simulink model "test_VirtualTestRig"  (R2021b)
settings: Solver=VariableStepAuto  StartTime=0.0  StopTime=10.0  RelTol=1e-3
settings Model: Creator=davide  LastModifiedBy=davide

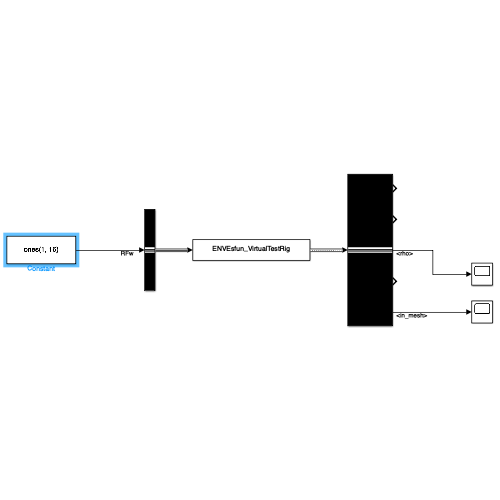
[thumbnail: Simulink's stored preview of the top-level diagram]
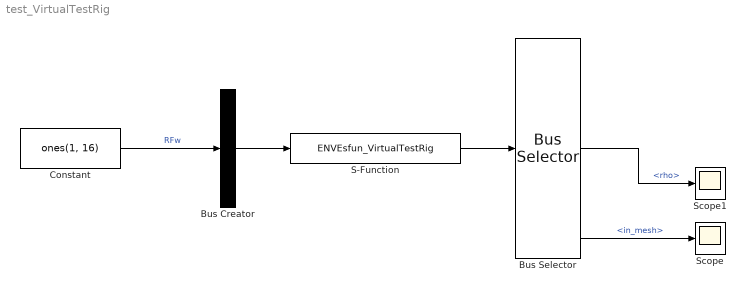
== system test_VirtualTestRig ==
  Bus Creator : BusCreator  Inputs=1  OutDataTypeStr=Bus: shellRF
  Bus Selector : BusSelector  OutputSignals=RFpc_ground,friction,rho,rho_dot,in_mesh
  Constant : Constant  Value=ones(1, 16)
  S-Function : S-Function  FunctionName=ENVEsfun_VirtualTestRig  Parameters=p1, p2, p3, p4, p5, p6, p7, p8  SFunctionDeploymentMode=off  EnableBusSupport=off
  Scope : Scope
  Scope1 : Scope
  wires:
  Bus Creator/1 -> S-Function/1
  S-Function/1 -> Bus Selector/1
  Constant/1 -> Bus Creator/1  "RFw"
  Bus Selector/5 -> Scope/1  "<in_mesh>"
  Bus Selector/3 -> Scope1/1  "<rho>"
